simulink model "IEEE24bus"  (R2019b)
settings: Solver=VariableStepAuto  StartTime=0.0  StopTime=100  RelTol=1e-3
values from neighbouring files (symbols this model uses):
  C_b = 1/(w_b*Z_b)    (= 5.01433343075e-06)    [IEEE24_bus.m]
  Exc = [ 011	0	 200	0.02	1.12   0.5   0	0       0       0       0       0 ... (first row only)    [IEEE24_bus.m]
  G_data = [ 011	15.8 138	2.8	0.2     2.7	1.5     0.3     7.5     0.25	0.04	0.85	0.85	0.25	0.12	0 ... (first row only)    [IEEE24_bus.m]
  H011 = 4    [IEEE24_bus.m]
  H012 = 4    [IEEE24_bus.m]
  H013 = 4    [IEEE24_bus.m]
  H021 = 4    [IEEE24_bus.m]
  H022 = 4    [IEEE24_bus.m]
  H023 = 4    [IEEE24_bus.m]
  H024 = 4    [IEEE24_bus.m]
  H025 = 4    [IEEE24_bus.m]
  H026 = 4    [IEEE24_bus.m]
  H131 = 4    [IEEE24_bus.m]
  H132 = 4    [IEEE24_bus.m]
  H133 = 4    [IEEE24_bus.m]
  H134 = 4    [IEEE24_bus.m]
  H135 = 4    [IEEE24_bus.m]
  H151 = 4    [IEEE24_bus.m]
  H152 = 4    [IEEE24_bus.m]
  H153 = 4    [IEEE24_bus.m]
  H154 = 4    [IEEE24_bus.m]
  H161 = 4    [IEEE24_bus.m]
  H181 = 3.25    [IEEE24_bus.m]
  H211 = 4    [IEEE24_bus.m]
  H212 = 4    [IEEE24_bus.m]
  H213 = 4    [IEEE24_bus.m]
  H215 = 4    [IEEE24_bus.m]
  H216 = 4    [IEEE24_bus.m]
  H221 = 3.25    [IEEE24_bus.m]
  H231 = 4    [IEEE24_bus.m]
  H232 = 4    [IEEE24_bus.m]
  H233 = 4    [IEEE24_bus.m]
  H234 = 4    [IEEE24_bus.m]
  H235 = 4    [IEEE24_bus.m]
  L_b = Z_b/w_b    (= 1.40321608159)    [IEEE24_bus.m]
  PSSMODEL = 1    [IEEE24_bus.m]    (also in IEEE24bus_simplified_benchmark.m)
  Z_b = (V_b^2)/S_b    (= 529)    [IEEE24_bus.m]
undefined symbols (not defined in the file or in its folder): D1, Delta
libraries: powerlib x258, sps_avr x33, microgridLibrary x6
(part 1 of 6)
settings Model: SimulationMode=accelerator  Creator=mingj  LastModifiedBy=tmj89

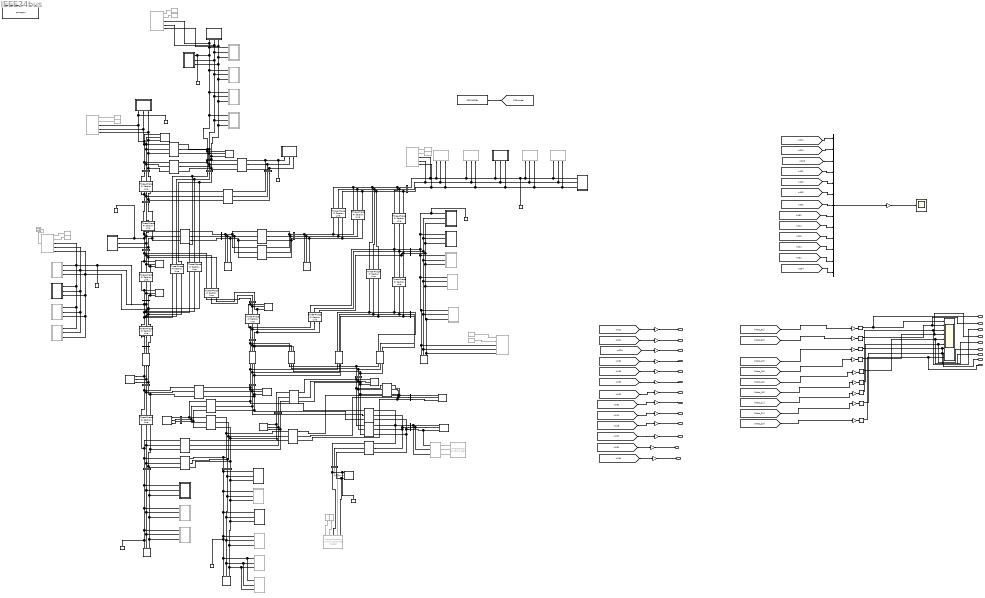
== system IEEE24bus ==
  011 : Subsystem
  012 : Subsystem  Commented=on
  013 : Subsystem  Commented=on
  "021 " : Subsystem
  022 : Subsystem  Commented=on
  023 : Subsystem
  024 : Subsystem  Commented=on
  025 : Subsystem  Commented=on
  026 : Subsystem  Commented=on
  1 : powerlib/Elements/Three-Phase PI Section Line  LConnTagsString=a|b|c  RConnTagsString=A|B|C  Frequency=60  Resistances="[0.00331*Z_b  0.00331*Z_b*3]"  Inductances="[0.02595*L_b  0.02595*L_b*3]"  Capacitances=[0.05330*C_b 0.05330*C_b/3]  Length=1
      settings: SourceProductName=Simscape Power Systems
  10 : powerlib/Elements/Three-Phase PI Section Line  LConnTagsString=a|b|c  RConnTagsString=A|B|C  Frequency=60  Resistances="[0.01224*Z_b  0.01224*Z_b*3]"  Inductances="[0.09644*L_b  0.09644*L_b*3]"  Capacitances=[0.1984*C_b 0.1984*C_b/3]  Length=1
      settings: SourceProductName=Simscape Power Systems
  11 : powerlib/Elements/Three-Phase PI Section Line  LConnTagsString=a|b|c  RConnTagsString=A|B|C  Frequency=60  Resistances="[0.01060*Z_b  0.01060*Z_b*3]"  Inductances="[0.08643*L_b  0.08643*L_b*3]"  Capacitances=[0.17520*C_b 0.17520*C_b/3]  Length=1
      settings: SourceProductName=Simscape Power Systems
  12 : powerlib/Elements/Three-Phase PI Section Line  LConnTagsString=a|b|c  RConnTagsString=A|B|C  Frequency=60  Resistances="[0.00583*Z_b  0.00583*Z_b*3]"  Inductances="[0.0476*L_b  0.0476*L_b*3]"  Capacitances=[0.0959*C_b 0.0959*C_b/3]  Length=1
      settings: SourceProductName=Simscape Power Systems
  131 : Subsystem
  132 : Subsystem
  133 : Subsystem  Commented=on
  134 : Subsystem  Commented=on
  135 : Subsystem  Commented=on
  14 : powerlib/Elements/Three-Phase PI Section Line  LConnTagsString=a|b|c  RConnTagsString=A|B|C  Frequency=60  Resistances="[0.00477*Z_b  0.00477*Z_b*3]"  Inductances="[0.03884*L_b  0.03884*L_b*3]"  Capacitances=[0.0785*C_b 0.0785*C_b/3]  Length=1
      settings: SourceProductName=Simscape Power Systems
  15 : powerlib/Elements/Three-Phase PI Section Line  LConnTagsString=a|b|c  RConnTagsString=A|B|C  Frequency=60  Resistances="[0.00513*Z_b  0.00513*Z_b*3]"  Inductances="[0.04172*L_b  0.04172*L_b*3]"  Capacitances=[0.0843*C_b 0.0843*C_b/3]  Length=1
      settings: SourceProductName=Simscape Power Systems
  151 : Subsystem  Commented=on
  152 : Subsystem
  153 : Subsystem  Commented=on
  154 : Subsystem  Commented=on
  16 : powerlib/Elements/Three-Phase PI Section Line  LConnTagsString=a|b|c  RConnTagsString=A|B|C  Frequency=60  Resistances="[0.00583*Z_b  0.00583*Z_b*3]"  Inductances="[0.04746*L_b  0.04746*L_b*3]"  Capacitances=[0.0959*C_b 0.0959*C_b/3]  Length=1
      settings: SourceProductName=Simscape Power Systems
  161 : Subsystem
  17 : powerlib/Elements/Three-Phase PI Section Line  LConnTagsString=a|b|c  RConnTagsString=A|B|C  Frequency=60  Resistances="[0.00642*Z_b  0.00642*Z_b*3]"  Inductances="[0.05187*L_b  0.05187*L_b*3]"  Capacitances=[0.1066*C_b 0.1066*C_b/3]  Length=1
      settings: SourceProductName=Simscape Power Systems
  18 : powerlib/Elements/Three-Phase PI Section Line  LConnTagsString=a|b|c  RConnTagsString=A|B|C  Frequency=60  Resistances="[0.05419*Z_b  0.05419*Z_b*3]"  Inductances="[0.21114*L_b  0.21114*L_b*3]"  Capacitances=[0.0613*C_b 0.0613*C_b/3]  Length=1
      settings: SourceProductName=Simscape Power Systems
  181 : Subsystem
  19 : powerlib/Elements/Three-Phase PI Section Line  LConnTagsString=a|b|c  RConnTagsString=A|B|C  Frequency=60  Resistances="[0.002*Z_b  0.002*Z_b*3]"  Inductances="[0.119*L_b  0.119*L_b*3]"  Capacitances=[0.0343*C_b 0.0343*C_b/3]  Length=1
      settings: SourceProductName=Simscape Power Systems
  2 : powerlib/Elements/Three-Phase PI Section Line  LConnTagsString=a|b|c  RConnTagsString=A|B|C  Frequency=60  Resistances="[0.00331*Z_b  0.00331*Z_b*3]"  Inductances="[0.02595*L_b  0.02595*L_b*3]"  Capacitances=[0.05330*C_b 0.05330*C_b/3]  Length=1
      settings: SourceProductName=Simscape Power Systems
  20 : powerlib/Elements/Three-Phase PI Section Line  LConnTagsString=a|b|c  RConnTagsString=A|B|C  Frequency=60  Resistances="[0.002*Z_b  0.002*Z_b*3]"  Inductances=[0.088*L_b 0.088*L_b*3]  Capacitances=[0.0478*C_b 0.0478*C_b/3]  Length=1
      settings: SourceProductName=Simscape Power Systems
  21 : powerlib/Elements/Three-Phase PI Section Line  LConnTagsString=a|b|c  RConnTagsString=A|B|C  Frequency=60  Resistances="[0.02692*Z_b  0.02692*Z_b*3]"  Inductances="[0.10779*L_b  0.10779*L_b*3]"  Capacitances=[0.0279*C_b 0.0279*C_b/3]  Length=1
      settings: SourceProductName=Simscape Power Systems
  211 : Subsystem
  212 : Subsystem  Commented=on
  213 : Subsystem  Commented=on
  214 : Subsystem  Commented=on
  215 : Subsystem  Commented=on
  216 : Subsystem
  22 : powerlib/Elements/Three-Phase PI Section Line  LConnTagsString=a|b|c  RConnTagsString=A|B|C  Frequency=60  Resistances=[0.03361*Z_b 0.03361*Z_b*3]  Inductances="[0.1273*L_b  0.1273*L_b*3]"  Capacitances=[0.0366*C_b 0.0366*C_b/3]  Length=1
      settings: SourceProductName=Simscape Power Systems
  221 : Subsystem
  23 : powerlib/Elements/Three-Phase PI Section Line  LConnTagsString=a|b|c  RConnTagsString=A|B|C  Frequency=60  Resistances="[0.02243*Z_b  0.02243*Z_b*3]"  Inductances=[0.0849*L_b 0.0849*L_b*3]  Capacitances=[0.0849*C_b 0.0849*C_b/3]  Length=1
      settings: SourceProductName=Simscape Power Systems
  231 : Subsystem
  232 : Subsystem  Commented=on
  233 : Subsystem  Commented=on
  234 : Subsystem
  235 : Subsystem  Commented=on
  236 : Subsystem  Commented=on
  24 : powerlib/Elements/Three-Phase PI Section Line  LConnTagsString=a|b|c  RConnTagsString=A|B|C  Frequency=60  Resistances="[0.0025*Z_b  0.0025*Z_b*3]"  Inductances="[0.014*L_b  0.014*L_b*3]"  Capacitances=[0.00065*C_b 0.00065*C_b/3]  Length=1
      settings: SourceProductName=Simscape Power Systems
  25 : powerlib/Elements/Three-Phase PI Section Line  LConnTagsString=a|b|c  RConnTagsString=A|B|C  Frequency=60  Resistances="[0.00607*Z_b  0.00607*Z_b*3]"  Inductances="[0.04899*L_b  0.04899*L_b*3]"  Capacitances=[0.10060*C_b 0.10060*C_b/3]  Length=1
      settings: SourceProductName=Simscape Power Systems
  26 : powerlib/Elements/Three-Phase PI Section Line  LConnTagsString=a|b|c  RConnTagsString=A|B|C  Frequency=60  Resistances="[0.05064*Z_b  0.05064*Z_b*3]"  Inductances="[0.19201*L_b  0.19201*L_b*3]"  Capacitances=[0.0557*C_b 0.0557*C_b/3]  Length=1
      settings: SourceProductName=Simscape Power Systems
  27 : powerlib/Elements/Three-Phase PI Section Line  LConnTagsString=a|b|c  RConnTagsString=A|B|C  Frequency=60  Resistances="[0.02262*Z_b  0.02262*Z_b*3]"  Inductances="[0.03333*L_b  0.03333*L_b*3]"  Capacitances=[0.13029*C_b 0.13029*C_b/3]  Length=1
      settings: SourceProductName=Simscape Power Systems
  28 : powerlib/Elements/Three-Phase PI Section Line  LConnTagsString=a|b|c  RConnTagsString=A|B|C  Frequency=60  Resistances="[0.00318*Z_b  0.00318*Z_b*3]"  Inductances="[0.025920*L_b  0.025920*L_b*3]"  Capacitances=[0.05230*C_b 0.05230*C_b/3]  Length=1
      settings: SourceProductName=Simscape Power Systems
  29 : powerlib/Elements/Three-Phase PI Section Line  LConnTagsString=a|b|c  RConnTagsString=A|B|C  Frequency=60  Resistances="[0.04234*Z_b  0.04234*Z_b*3]"  Inductances="[0.16482*L_b  0.16482*L_b*3]"  Capacitances=[0.0478*C_b 0.0478*C_b/3]  Length=1
      settings: SourceProductName=Simscape Power Systems
  3 : powerlib/Elements/Three-Phase PI Section Line  LConnTagsString=a|b|c  RConnTagsString=A|B|C  Frequency=60  Resistances="[0.00829*Z_b  0.00829*Z_b*3]"  Inductances="[0.06769*L_b  0.06769*L_b*3]"  Capacitances=[0.13670*C_b 0.13670*C_b/3]  Length=1
      settings: SourceProductName=Simscape Power Systems
  3-Phase Dynamic Load3 : powerlib/Elements/Three-Phase Dynamic Load  Commented=on  NominalVoltage=[ 20e3 60 ]  ActiveReactivePowers=[-1e6 -1e6]  PositiveSequence=[0.999196 -2.87767]  ExternalControl=off  NpNq="[0  0]"  TimeConstants=[0 0 0 0]  MinimumVoltage=0.01  Tfilter=1e-1  LoadFlowParameters=[4 50000000 0 0 25000000]
      settings: SourceProductName=Simscape Power Systems  SourceProductBaseCode=PS
  30 : powerlib/Elements/Three-Phase PI Section Line  LConnTagsString=a|b|c  RConnTagsString=A|B|C  Frequency=60  Resistances="[0.00177*Z_b  0.00177*Z_b*3]"  Inductances="[0.01439*L_b  0.01439*L_b*3]"  Capacitances=[0.02910*C_b 0.02910*C_b/3]  Length=1
      settings: SourceProductName=Simscape Power Systems
  31 : powerlib/Elements/Three-Phase PI Section Line  LConnTagsString=a|b|c  RConnTagsString=A|B|C  Frequency=60  Resistances="[0.04234*Z_b  0.04234*Z_b*3]"  Inductances="[0.16482*L_b  0.16482*L_b*3]"  Capacitances=[0.0478*C_b 0.0478*C_b/3]  Length=1
      settings: SourceProductName=Simscape Power Systems
  32 : powerlib/Elements/Three-Phase PI Section Line  LConnTagsString=a|b|c  RConnTagsString=A|B|C  Frequency=60  Resistances=[0.01614*Z_b 0.01614*Z_b*3]  Inductances="[0.06103*L_b  0.06103*L_b*3]"  Capacitances=[0.0179*C_b 0.0179*C_b/3]  Length=1
      settings: SourceProductName=Simscape Power Systems
  4 : powerlib/Elements/Three-Phase PI Section Line  LConnTagsString=a|b|c  RConnTagsString=A|B|C  Frequency=60  Resistances="[0.01225*Z_b  0.01225*Z_b*3]"  Inductances="[0.10527*L_b  0.10527*L_b*3]"  Capacitances=[0.21160*C_b 0.21160*C_b/3]  Length=1
      settings: SourceProductName=Simscape Power Systems
  43 : powerlib/Elements/Three-Phase PI Section Line  LConnTagsString=a|b|c  RConnTagsString=A|B|C  Frequency=60  Resistances=[0.00607*Z_b 0.00607*Z_b*3]  Inductances="[0.04899*L_b  0.04899*L_b*3]"  Capacitances=[0.10060*C_b 0.10060*C_b/3]  Length=1
      settings: SourceProductName=Simscape Power Systems
  5 : powerlib/Elements/Three-Phase PI Section Line  LConnTagsString=a|b|c  RConnTagsString=A|B|C  Frequency=60  Resistances="[0.00283*Z_b  0.00283*Z_b*3]"  Inductances="[0.02302*L_b  0.02302*L_b*3]"  Capacitances=[0.04650*C_b 0.04650*C_b/3]  Length=1
      settings: SourceProductName=Simscape Power Systems
  6 : powerlib/Elements/Three-Phase PI Section Line  LConnTagsString=a|b|c  RConnTagsString=A|B|C  Frequency=60  Resistances="[0.00505*Z_b  0.00505*Z_b*3]"  Inductances="[0.03964*L_b  0.03964*L_b*3]"  Capacitances=[0.08140*C_b 0.08140*C_b/3]  Length=1
      settings: SourceProductName=Simscape Power Systems
  7 : powerlib/Elements/Three-Phase PI Section Line  LConnTagsString=a|b|c  RConnTagsString=A|B|C  Frequency=60  Resistances="[0.00505*Z_b  0.00505*Z_b*3]"  Inductances="[0.03964*L_b  0.03964*L_b*3]"  Capacitances=[0.08140*C_b 0.08140*C_b/3]  Length=1
      settings: SourceProductName=Simscape Power Systems
  8 : powerlib/Elements/Three-Phase PI Section Line  LConnTagsString=a|b|c  RConnTagsString=A|B|C  Frequency=60  Resistances="[0.00276*Z_b  0.00276*Z_b*3]"  Inductances="[0.02163*L_b  0.02163*L_b*3]"  Capacitances=[0.04440*C_b 0.04440*C_b/3]  Length=1
      settings: SourceProductName=Simscape Power Systems
  9 : powerlib/Elements/Three-Phase PI Section Line  LConnTagsString=a|b|c  RConnTagsString=A|B|C  Frequency=60  Resistances="[0.00276*Z_b  0.00276*Z_b*3]"  Inductances="[0.02163*L_b  0.02163*L_b*3]"  Capacitances=[0.04440*C_b 0.04440*C_b/3]  Length=1
      settings: SourceProductName=Simscape Power Systems
  Base Load 1 : powerlib/Elements/Three-Phase Parallel RLC Load  LConnTagsString=A|B|C  Configuration=Y (grounded)  NominalVoltage=230e3  Vabc=[1e3 1e3 1e3]  Vabcp=[1e3 1e3 1e3]  NominalFrequency=60  UnbalancedPower=off  ActivePower=L19  InductivePower=18e6  CapacitivePower=0  Pabc=[10e3 9e3 11e3]  QLabc=[100 90 110]  QCabc=[100 90 110]  Pabcp=[10e3 9e3 11e3]  QLabcp=[100 90 110]  QCabcp=[100 90 110]  Measurements=None  LoadType=constant Z
      settings: SourceProductName=Simscape Electrical
  Base Load 10 : powerlib/Elements/Three-Phase Parallel RLC Load  LConnTagsString=A|B|C  Configuration=Y (grounded)  NominalVoltage=138e3  Vabc=[1e3 1e3 1e3]  Vabcp=[1e3 1e3 1e3]  NominalFrequency=60  UnbalancedPower=off  ActivePower=L1  InductivePower=22e6  CapacitivePower=0  Pabc=[10e3 9e3 11e3]  QLabc=[100 90 110]  QCabc=[100 90 110]  Pabcp=[10e3 9e3 11e3]  QLabcp=[100 90 110]  QCabcp=[100 90 110]  Measurements=None  LoadType=constant Z
      settings: SourceProductName=Simscape Electrical
  Base Load 11 : powerlib/Elements/Three-Phase Parallel RLC Load  LConnTagsString=A|B|C  Configuration=Y (grounded)  NominalVoltage=138e3  Vabc=[1e3 1e3 1e3]  Vabcp=[1e3 1e3 1e3]  NominalFrequency=60  UnbalancedPower=off  ActivePower=L2  InductivePower=20e6  CapacitivePower=0  Pabc=[10e3 9e3 11e3]  QLabc=[100 90 110]  QCabc=[100 90 110]  Pabcp=[10e3 9e3 11e3]  QLabcp=[100 90 110]  QCabcp=[100 90 110]  Measurements=None  LoadType=constant Z
      settings: SourceProductName=Simscape Electrical
  Base Load 12 : powerlib/Elements/Three-Phase Parallel RLC Load  LConnTagsString=A|B|C  Configuration=Y (grounded)  NominalVoltage=138e3  Vabc=[1e3 1e3 1e3]  Vabcp=[1e3 1e3 1e3]  NominalFrequency=60  UnbalancedPower=off  ActivePower=L3  InductivePower=19e6  CapacitivePower=0  Pabc=[10e3 9e3 11e3]  QLabc=[100 90 110]  QCabc=[100 90 110]  Pabcp=[10e3 9e3 11e3]  QLabcp=[100 90 110]  QCabcp=[100 90 110]  Measurements=None  LoadType=constant Z
      settings: SourceProductName=Simscape Electrical
  Base Load 13 : powerlib/Elements/Three-Phase Parallel RLC Load  LConnTagsString=A|B|C  Configuration=Y (grounded)  NominalVoltage=138e3  Vabc=[1e3 1e3 1e3]  Vabcp=[1e3 1e3 1e3]  NominalFrequency=60  UnbalancedPower=off  ActivePower=L5  InductivePower=14e6  CapacitivePower=0  Pabc=[10e3 9e3 11e3]  QLabc=[100 90 110]  QCabc=[100 90 110]  Pabcp=[10e3 9e3 11e3]  QLabcp=[100 90 110]  QCabcp=[100 90 110]  Measurements=None  LoadType=constant Z
      settings: SourceProductName=Simscape Electrical
  Base Load 14 : powerlib/Elements/Three-Phase Parallel RLC Load  LConnTagsString=A|B|C  Configuration=Y (grounded)  NominalVoltage=230e3  Vabc=[1e3 1e3 1e3]  Vabcp=[1e3 1e3 1e3]  NominalFrequency=60  UnbalancedPower=off  ActivePower=L13  InductivePower=27e6  CapacitivePower=0  Pabc=[10e3 9e3 11e3]  QLabc=[100 90 110]  QCabc=[100 90 110]  Pabcp=[10e3 9e3 11e3]  QLabcp=[100 90 110]  QCabcp=[100 90 110]  Measurements=None  LoadType=constant Z
      settings: SourceProductName=Simscape Electrical
  Base Load 15 : powerlib/Elements/Three-Phase Parallel RLC Load  LConnTagsString=A|B|C  Configuration=Y (grounded)  NominalVoltage=230e3  Vabc=[1e3 1e3 1e3]  Vabcp=[1e3 1e3 1e3]  NominalFrequency=60  UnbalancedPower=off  ActivePower=L14  InductivePower=20e6  CapacitivePower=0  Pabc=[10e3 9e3 11e3]  QLabc=[100 90 110]  QCabc=[100 90 110]  Pabcp=[10e3 9e3 11e3]  QLabcp=[100 90 110]  QCabcp=[100 90 110]  Measurements=None  LoadType=constant Z
      settings: SourceProductName=Simscape Electrical
  Base Load 16 : powerlib/Elements/Three-Phase Parallel RLC Load  LConnTagsString=A|B|C  Configuration=Y (grounded)  NominalVoltage=230e3  Vabc=[1e3 1e3 1e3]  Vabcp=[1e3 1e3 1e3]  NominalFrequency=60  UnbalancedPower=off  ActivePower=L15  InductivePower=32e6  CapacitivePower=0  Pabc=[10e3 9e3 11e3]  QLabc=[100 90 110]  QCabc=[100 90 110]  Pabcp=[10e3 9e3 11e3]  QLabcp=[100 90 110]  QCabcp=[100 90 110]  Measurements=None  LoadType=constant Z
      settings: SourceProductName=Simscape Electrical
  Base Load 17 : powerlib/Elements/Three-Phase Parallel RLC Load  LConnTagsString=A|B|C  Configuration=Y (grounded)  NominalVoltage=230e3  Vabc=[1e3 1e3 1e3]  Vabcp=[1e3 1e3 1e3]  NominalFrequency=60  UnbalancedPower=off  ActivePower=L16  InductivePower=0  CapacitivePower=0  Pabc=[10e3 9e3 11e3]  QLabc=[100 90 110]  QCabc=[100 90 110]  Pabcp=[10e3 9e3 11e3]  QLabcp=[100 90 110]  QCabcp=[100 90 110]  Measurements=None  LoadType=constant Z
      settings: SourceProductName=Simscape Electrical
  Base Load 18 : powerlib/Elements/Three-Phase Parallel RLC Load  LConnTagsString=A|B|C  Configuration=Y (grounded)  NominalVoltage=230e3  Vabc=[1e3 1e3 1e3]  Vabcp=[1e3 1e3 1e3]  NominalFrequency=60  UnbalancedPower=off  ActivePower=L21  InductivePower=34e6  CapacitivePower=0  Pabc=[10e3 9e3 11e3]  QLabc=[100 90 110]  QCabc=[100 90 110]  Pabcp=[10e3 9e3 11e3]  QLabcp=[100 90 110]  QCabcp=[100 90 110]  Measurements=None  LoadType=constant Z
      settings: SourceProductName=Simscape Electrical
  Base Load 2 : powerlib/Elements/Three-Phase Parallel RLC Load  LConnTagsString=A|B|C  Configuration=Y (grounded)  NominalVoltage=230e3  Vabc=[1e3 1e3 1e3]  Vabcp=[1e3 1e3 1e3]  NominalFrequency=60  UnbalancedPower=off  ActivePower=L20  InductivePower=13e6  CapacitivePower=0  Pabc=[10e3 9e3 11e3]  QLabc=[100 90 110]  QCabc=[100 90 110]  Pabcp=[10e3 9e3 11e3]  QLabcp=[100 90 110]  QCabcp=[100 90 110]  Measurements=None  LoadType=constant Z
      settings: SourceProductName=Simscape Electrical
  Base Load 3 : powerlib/Elements/Three-Phase Parallel RLC Load  LConnTagsString=A|B|C  Configuration=Y (grounded)  NominalVoltage=138e3  Vabc=[1e3 1e3 1e3]  Vabcp=[1e3 1e3 1e3]  NominalFrequency=60  UnbalancedPower=off  ActivePower=L6  InductivePower=14e6  CapacitivePower=0  Pabc=[10e3 9e3 11e3]  QLabc=[100 90 110]  QCabc=[100 90 110]  Pabcp=[10e3 9e3 11e3]  QLabcp=[100 90 110]  QCabcp=[100 90 110]  Measurements=None  LoadType=constant Z
      settings: SourceProductName=Simscape Electrical
  Base Load 4 : powerlib/Elements/Three-Phase Parallel RLC Load  LConnTagsString=A|B|C  Configuration=Y (grounded)  NominalVoltage=138e3  Vabc=[1e3 1e3 1e3]  Vabcp=[1e3 1e3 1e3]  NominalFrequency=60  UnbalancedPower=off  ActivePower=L8  InductivePower=18e6  CapacitivePower=0  Pabc=[10e3 9e3 11e3]  QLabc=[100 90 110]  QCabc=[100 90 110]  Pabcp=[10e3 9e3 11e3]  QLabcp=[100 90 110]  QCabcp=[100 90 110]  Measurements=None  LoadType=constant Z
      settings: SourceProductName=Simscape Electrical
  Base Load 5 : powerlib/Elements/Three-Phase Parallel RLC Load  LConnTagsString=A|B|C  Configuration=Y (grounded)  NominalVoltage=230e3  Vabc=[1e3 1e3 1e3]  Vabcp=[1e3 1e3 1e3]  NominalFrequency=60  UnbalancedPower=off  ActivePower=L18  InductivePower=34e6  CapacitivePower=0  Pabc=[10e3 9e3 11e3]  QLabc=[100 90 110]  QCabc=[100 90 110]  Pabcp=[10e3 9e3 11e3]  QLabcp=[100 90 110]  QCabcp=[100 90 110]  Measurements=None  LoadType=constant Z
      settings: SourceProductName=Simscape Electrical
  Base Load 6 : powerlib/Elements/Three-Phase Parallel RLC Load  LConnTagsString=A|B|C  Configuration=Y (grounded)  NominalVoltage=138e3  Vabc=[1e3 1e3 1e3]  Vabcp=[1e3 1e3 1e3]  NominalFrequency=60  UnbalancedPower=off  ActivePower=L4  InductivePower=15e6  CapacitivePower=0  Pabc=[10e3 9e3 11e3]  QLabc=[100 90 110]  QCabc=[100 90 110]  Pabcp=[10e3 9e3 11e3]  QLabcp=[100 90 110]  QCabcp=[100 90 110]  Measurements=None  LoadType=constant Z
      settings: SourceProductName=Simscape Electrical
  Base Load 7 : powerlib/Elements/Three-Phase Parallel RLC Load  LConnTagsString=A|B|C  Configuration=Y (grounded)  NominalVoltage=138e3  Vabc=[1e3 1e3 1e3]  Vabcp=[1e3 1e3 1e3]  NominalFrequency=60  UnbalancedPower=off  ActivePower=L9  InductivePower=36e6  CapacitivePower=0  Pabc=[10e3 9e3 11e3]  QLabc=[100 90 110]  QCabc=[100 90 110]  Pabcp=[10e3 9e3 11e3]  QLabcp=[100 90 110]  QCabcp=[100 90 110]  Measurements=None  LoadType=constant Z
      settings: SourceProductName=Simscape Electrical
  Base Load 8 : powerlib/Elements/Three-Phase Parallel RLC Load  LConnTagsString=A|B|C  Configuration=Y (grounded)  NominalVoltage=138e3  Vabc=[1e3 1e3 1e3]  Vabcp=[1e3 1e3 1e3]  NominalFrequency=60  UnbalancedPower=off  ActivePower=L10  InductivePower=23e6  CapacitivePower=0  Pabc=[10e3 9e3 11e3]  QLabc=[100 90 110]  QCabc=[100 90 110]  Pabcp=[10e3 9e3 11e3]  QLabcp=[100 90 110]  QCabcp=[100 90 110]  Measurements=None  LoadType=constant Z
      settings: SourceProductName=Simscape Electrical
  Base Load 9 : powerlib/Elements/Three-Phase Parallel RLC Load  LConnTagsString=A|B|C  Configuration=Y (grounded)  NominalVoltage=138e3  Vabc=[1e3 1e3 1e3]  Vabcp=[1e3 1e3 1e3]  NominalFrequency=60  UnbalancedPower=off  ActivePower=L7  InductivePower=13e6  CapacitivePower=0  Pabc=[10e3 9e3 11e3]  QLabc=[100 90 110]  QCabc=[100 90 110]  Pabcp=[10e3 9e3 11e3]  QLabcp=[100 90 110]  QCabcp=[100 90 110]  Measurements=None  LoadType=constant Z
      settings: SourceProductName=Simscape Electrical
  Bus1 : powerlib/Measurements/Three-Phase V-I Measurement  VoltageMeasurement=phase-to-phase  SetLabelV=on  LabelV=Vabc_01  Vpu=on  VpuLL=off  CurrentMeasurement=no  SetLabelI=on  LabelI=Iabc_1  Ipu=on  Pbase=S_b  Vbase=V_bl  OutputType=Complex  PhasorSimulation=on  PSBequivalent=0
      settings: SourceProductName=Simscape Electrical
  Bus{3..6,8..12,14,17,19,24} (13 alike) : powerlib/Measurements/Three-Phase V-I Measurement  VoltageMeasurement=no  SetLabelV=on  LabelV=Vabc_1  Vpu=on  VpuLL=off  CurrentMeasurement=no  SetLabelI=on  LabelI=Iabc_1  Ipu=on  Pbase=S_b  Vbase=V_b  OutputType=Complex  PhasorSimulation=on  PSBequivalent=0
      settings: SourceProductName=Simscape Electrical
  Bus13 : powerlib/Measurements/Three-Phase V-I Measurement  VoltageMeasurement=phase-to-phase  SetLabelV=on  LabelV=Vabc_13  Vpu=on  VpuLL=off  CurrentMeasurement=no  SetLabelI=on  LabelI=Iabc_1  Ipu=on  Pbase=S_b  Vbase=V_b  OutputType=Complex  PhasorSimulation=on  PSBequivalent=0
      settings: SourceProductName=Simscape Electrical
  Bus15 : powerlib/Measurements/Three-Phase V-I Measurement  VoltageMeasurement=phase-to-phase  SetLabelV=on  LabelV=Vabc_15  Vpu=on  VpuLL=off  CurrentMeasurement=no  SetLabelI=on  LabelI=Iabc_1  Ipu=on  Pbase=S_b  Vbase=V_b  OutputType=Complex  PhasorSimulation=on  PSBequivalent=0
      settings: SourceProductName=Simscape Electrical
  Bus16 : powerlib/Measurements/Three-Phase V-I Measurement  VoltageMeasurement=phase-to-phase  SetLabelV=on  LabelV=Vabc_16  Vpu=on  VpuLL=off  CurrentMeasurement=no  SetLabelI=on  LabelI=Iabc_1  Ipu=on  Pbase=S_b  Vbase=V_b  OutputType=Complex  PhasorSimulation=on  PSBequivalent=0
      settings: SourceProductName=Simscape Electrical
  Bus18 : powerlib/Measurements/Three-Phase V-I Measurement  VoltageMeasurement=phase-to-phase  SetLabelV=on  LabelV=Vabc_18  Vpu=on  VpuLL=off  CurrentMeasurement=no  SetLabelI=on  LabelI=Iabc_1  Ipu=on  Pbase=S_b  Vbase=V_b  OutputType=Complex  PhasorSimulation=on  PSBequivalent=0
      settings: SourceProductName=Simscape Electrical
  Bus2 : powerlib/Measurements/Three-Phase V-I Measurement  VoltageMeasurement=phase-to-phase  SetLabelV=on  LabelV=Vabc_02  Vpu=on  VpuLL=off  CurrentMeasurement=no  SetLabelI=on  LabelI=Iabc_1  Ipu=on  Pbase=S_b  Vbase=V_bl  OutputType=Complex  PhasorSimulation=on  PSBequivalent=0
      settings: SourceProductName=Simscape Electrical
  Bus20 : powerlib/Measurements/Three-Phase V-I Measurement  VoltageMeasurement=no  SetLabelV=on  LabelV=Vabc_20  Vpu=on  VpuLL=off  CurrentMeasurement=yes  SetLabelI=on  LabelI=Iabc_20  Ipu=on  Pbase=S_b  Vbase=V_b  OutputType=Complex  PhasorSimulation=on  PSBequivalent=0
      settings: SourceProductName=Simscape Electrical
  Bus21 : powerlib/Measurements/Three-Phase V-I Measurement  VoltageMeasurement=phase-to-phase  SetLabelV=on  LabelV=Vabc_21  Vpu=on  VpuLL=off  CurrentMeasurement=no  SetLabelI=on  LabelI=Iabc_1  Ipu=on  Pbase=S_b  Vbase=V_b  OutputType=Complex  PhasorSimulation=on  PSBequivalent=0
      settings: SourceProductName=Simscape Electrical
  Bus22 : powerlib/Measurements/Three-Phase V-I Measurement  VoltageMeasurement=phase-to-phase  SetLabelV=on  LabelV=Vabc_22  Vpu=on  VpuLL=off  CurrentMeasurement=no  SetLabelI=on  LabelI=Iabc_1  Ipu=on  Pbase=S_b  Vbase=V_b  OutputType=Complex  PhasorSimulation=on  PSBequivalent=0
      settings: SourceProductName=Simscape Electrical
  Bus23 : powerlib/Measurements/Three-Phase V-I Measurement  VoltageMeasurement=phase-to-phase  SetLabelV=on  LabelV=Vabc_23  Vpu=on  VpuLL=off  CurrentMeasurement=no  SetLabelI=on  LabelI=Iabc_1  Ipu=on  Pbase=S_b  Vbase=V_b  OutputType=Complex  PhasorSimulation=on  PSBequivalent=0
      settings: SourceProductName=Simscape Electrical
  Bus7 : powerlib/Measurements/Three-Phase V-I Measurement  VoltageMeasurement=phase-to-phase  SetLabelV=on  LabelV=Vabc_07  Vpu=on  VpuLL=off  CurrentMeasurement=no  SetLabelI=on  LabelI=Iabc_1  Ipu=on  Pbase=S_b  Vbase=V_bl  OutputType=Complex  PhasorSimulation=on  PSBequivalent=0
      settings: SourceProductName=Simscape Electrical
  CPS mag : Scope  NumInputPorts=9
  Constant{8,10,13,19,25,27} (6 alike) : Constant  Commented=on  Value=0
  Constant{9,11,14,20,26,28} (6 alike) : Constant  Commented=on  Value=15
  Gain{,1..8} (9 alike) : Gain  Gain=[1 0 0]  Multiplication=Matrix(K*u) (u vector)
  L-49-2 : powerlib/Elements/Three-Phase PI Section Line  LConnTagsString=a|b|c  RConnTagsString=A|B|C  Frequency=60  Resistances="[0.00212*Z_b  0.00212*Z_b*3]"  Inductances="[ 0.17269*L_b  0.17269*L_b*3]"  Capacitances=[ 0.03490*C_b 0.03490*C_b/3]  Length=1
      settings: SourceProductName=Simscape Power Systems
  Load Flow Bus : powerlib/Measurements/Load Flow Bus  LConnTagsString=a  Phases=single  Connectors=on one side  ID=BUS_18  Vbase=230e3  Vref=1.05  Vangle=0  VLF=0.975  VLFb=1  VLFc=1  angleLF=48.06  angleLFb=0  angleLFc=0
      settings: AttributesFormatString=%<ID>\n%<Vbase>V\n%<VLF>pu\n%<angleLF>deg.  SourceProductName=Simscape Electrical
  Load Flow Bus1 : powerlib/Measurements/Load Flow Bus  LConnTagsString=a  Phases=single  Connectors=on one side  ID=BUS_02  Vbase=138e3  Vref=1.035  Vangle=0  VLF=1.001  VLFb=1  VLFc=1  angleLF=21.1  angleLFb=0  angleLFc=0
      settings: AttributesFormatString=%<ID>\n%<Vbase>V\n%<VLF>pu\n%<angleLF>deg.  SourceProductName=Simscape Electrical
  Load Flow Bus10 : powerlib/Measurements/Load Flow Bus  LConnTagsString=a  Phases=single  Connectors=on one side  ID=BUS_13  Vbase=230e3  Vref=1.02  Vangle=0  VLF=0.9742  VLFb=1  VLFc=1  angleLF=29.58  angleLFb=0  angleLFc=0
      settings: AttributesFormatString=%<ID>\n%<Vbase>V\n%<VLF>pu\n%<angleLF>deg.  SourceProductName=Simscape Electrical
  Load Flow Bus11 : powerlib/Measurements/Load Flow Bus  LConnTagsString=a  Phases=single  Connectors=on one side  ID=BUS_16  Vbase=230e3  Vref=1.017  Vangle=0  VLF=0.9617  VLFb=1  VLFc=1  angleLF=41.74  angleLFb=0  angleLFc=0
      settings: AttributesFormatString=%<ID>\n%<Vbase>V\n%<VLF>pu\n%<angleLF>deg.  SourceProductName=Simscape Electrical
  Load Flow Bus2 : powerlib/Measurements/Load Flow Bus  LConnTagsString=a  Phases=single  Connectors=on one side  ID=BUS_07  Vbase=138e3  Vref=1.025  Vangle=0  VLF=0.9748  VLFb=1  VLFc=1  angleLF=21.22  angleLFb=0  angleLFc=0
      settings: AttributesFormatString=%<ID>\n%<Vbase>V\n%<VLF>pu\n%<angleLF>deg.  SourceProductName=Simscape Electrical
  Load Flow Bus3 : powerlib/Measurements/Load Flow Bus  LConnTagsString=a  Phases=single  Connectors=on one side  ID=BUS_21  Vbase=230e3  Vref=1.05  Vangle=0  VLF=0.9792  VLFb=1  VLFc=1  angleLF=48.86  angleLFb=0  angleLFc=0
      settings: AttributesFormatString=%<ID>\n%<Vbase>V\n%<VLF>pu\n%<angleLF>deg.  SourceProductName=Simscape Electrical
  Load Flow Bus4 : powerlib/Measurements/Load Flow Bus  LConnTagsString=a  Phases=single  Connectors=on one side  ID=BUS_01  Vbase=138e3  Vref=1.035  Vangle=0  VLF=0.9978  VLFb=1  VLFc=1  angleLF=21.25  angleLFb=0  angleLFc=0
      settings: AttributesFormatString=%<ID>\n%<Vbase>V\n%<VLF>pu\n%<angleLF>deg.  SourceProductName=Simscape Electrical
  Load Flow Bus5 : powerlib/Measurements/Load Flow Bus  LConnTagsString=a  Phases=single  Connectors=on one side  ID=BUS_15  Vbase=230e3  Vref=1.014  Vangle=0  VLF=0.9593  VLFb=1  VLFc=1  angleLF=42.73  angleLFb=0  angleLFc=0
      settings: AttributesFormatString=%<ID>\n%<Vbase>V\n%<VLF>pu\n%<angleLF>deg.  SourceProductName=Simscape Electrical
  Load Flow Bus6 : powerlib/Measurements/Load Flow Bus  LConnTagsString=a  Phases=single  Connectors=on one side  ID=BUS_22  Vbase=230e3  Vref=1.05  Vangle=0  VLF=0.9939  VLFb=1  VLFc=1  angleLF=55.21  angleLFb=0  angleLFc=0
      settings: AttributesFormatString=%<ID>\n%<Vbase>V\n%<VLF>pu\n%<angleLF>deg.  SourceProductName=Simscape Electrical
  Load Flow Bus7 : powerlib/Measurements/Load Flow Bus  LConnTagsString=a  Phases=single  Connectors=on one side  ID=BUS_23  Vbase=230e3  Vref=1.05  Vangle=0  VLF=0.9824  VLFb=1  VLFc=1  angleLF=41.99  angleLFb=0  angleLFc=0
      settings: AttributesFormatString=%<ID>\n%<Vbase>V\n%<VLF>pu\n%<angleLF>deg.  SourceProductName=Simscape Electrical
  Mux : Mux  Inputs=13
  PSS model : Constant  Value=PSSMODEL
  Power Equation Wind Turbine (PQ Model)10 : microgridLibrary/Power Equation Wind Turbine (PQ Model)  Commented=on  Unom=15  Umax=25  Umin=5  Pselect=Simple Cubic Power  Vrms=230*1e3  Fnom=60  rp=5  Cp=16/27  rho=1.225  Pnom=60*1e6  Uvec=[1:1:30]  Pvec=[0,0,0,0,21359.3750000000,58193.5000000000,104316.125000000,157104.500000000,213935.875000000,272187.500000000,329236.625000000,382460.500000000,429236.375000000,466941.500000000,492953.125000000,500000,500000,500000,500000,500000,500000,500000,500000,500000,500000,0,0,0,0,0]  Tp=0.1  Tq=1  ReactP=0
  Power Equation Wind Turbine (PQ Model)11 : microgridLibrary/Power Equation Wind Turbine (PQ Model)  Commented=on  Unom=15  Umax=25  Umin=5  Pselect=Simple Cubic Power  Vrms=138*1e3  Fnom=60  rp=5  Cp=16/27  rho=1.225  Pnom=50e6  Uvec=[1:1:30]  Pvec=[0,0,0,0,21359.3750000000,58193.5000000000,104316.125000000,157104.500000000,213935.875000000,272187.500000000,329236.625000000,382460.500000000,429236.375000000,466941.500000000,492953.125000000,500000,500000,500000,500000,500000,500000,500000,500000,500000,500000,0,0,0,0,0]  Tp=0.1  Tq=1  ReactP=0
  Power Equation Wind Turbine (PQ Model)12 : microgridLibrary/Power Equation Wind Turbine (PQ Model)  Commented=on  Unom=15  Umax=25  Umin=5  Pselect=Simple Cubic Power  Vrms=230*1e3  Fnom=60  rp=5  Cp=16/27  rho=1.225  Pnom=160e6  Uvec=[1:1:30]  Pvec=[0,0,0,0,21359.3750000000,58193.5000000000,104316.125000000,157104.500000000,213935.875000000,272187.500000000,329236.625000000,382460.500000000,429236.375000000,466941.500000000,492953.125000000,500000,500000,500000,500000,500000,500000,500000,500000,500000,500000,0,0,0,0,0]  Tp=0.1  Tq=1  ReactP=0
  Power Equation Wind Turbine (PQ Model)13 : microgridLibrary/Power Equation Wind Turbine (PQ Model)  Commented=on  Unom=15  Umax=25  Umin=5  Pselect=Simple Cubic Power  Vrms=230*1e3  Fnom=60  rp=5  Cp=16/27  rho=1.225  Pnom=300*1e6  Uvec=[1:1:30]  Pvec=[0,0,0,0,21359.3750000000,58193.5000000000,104316.125000000,157104.500000000,213935.875000000,272187.500000000,329236.625000000,382460.500000000,429236.375000000,466941.500000000,492953.125000000,500000,500000,500000,500000,500000,500000,500000,500000,500000,500000,0,0,0,0,0]  Tp=0.1  Tq=1  ReactP=0
  Power Equation Wind Turbine (PQ Model)8 : microgridLibrary/Power Equation Wind Turbine (PQ Model)  Commented=on  Unom=15  Umax=25  Umin=5  Pselect=Simple Cubic Power  Vrms=230*1e3  Fnom=60  rp=5  Cp=16/27  rho=1.225  Pnom=60*1e6  Uvec=[1:1:30]  Pvec=[0,0,0,0,21359.3750000000,58193.5000000000,104316.125000000,157104.500000000,213935.875000000,272187.500000000,329236.625000000,382460.500000000,429236.375000000,466941.500000000,492953.125000000,500000,500000,500000,500000,500000,500000,500000,500000,500000,500000,0,0,0,0,0]  Tp=0.1  Tq=1  ReactP=0
  Power Equation Wind Turbine (PQ Model)9 : microgridLibrary/Power Equation Wind Turbine (PQ Model)  Commented=on  Unom=15  Umax=25  Umin=5  Pselect=Simple Cubic Power  Vrms=230*1e3  Fnom=60  rp=5  Cp=16/27  rho=1.225  Pnom=60*1e6  Uvec=[1:1:30]  Pvec=[0,0,0,0,21359.3750000000,58193.5000000000,104316.125000000,157104.500000000,213935.875000000,272187.500000000,329236.625000000,382460.500000000,429236.375000000,466941.500000000,492953.125000000,500000,500000,500000,500000,500000,500000,500000,500000,500000,500000,0,0,0,0,0]  Tp=0.1  Tq=1  ReactP=0
  Scope1 : Scope  Commented=on
  TVI4 : powerlib/Elements/Three-Phase Transformer (Two Windings)  Commented=on  Winding1Connection=Yg  Winding2Connection=Yg  CoreType=Three single-phase transformers  SetSaturation=off  Hysteresis=off  DataFile='hysteresis'  SetInitialFlux=off  Measurements=None  UNITS=pu  NominalPower=[ 400*1e6 , 60 ]  Winding1=[ 20*1e3, 1e-6 , 0 ]  Winding2=[ 230*1e3, 0 , 17 ]  Rm=500  Lm=500  L0=0.5  Saturation=[ 0,0 ; 0.0024,1.2 ; 1.0,1.52 ]  InitialFluxes=[ 0.8 , -0.8 , 0.7 ]  BreakLoop=off  DiscreteSolver=Trapezoidal iterative  DataType=off  TransfoNumber=0
  Trafo 14 : powerlib/Elements/Three-Phase Transformer (Two Windings)  Winding1Connection=Delta (D1)  Winding2Connection=Yg  CoreType=Three single-phase transformers  SetSaturation=off  Hysteresis=off  DataFile='hysteresis'  SetInitialFlux=off  Measurements=None  UNITS=pu  NominalPower=[ 400e6 60 ]  Winding1="[138e3 0.0023  0.0839]"  Winding2=[230e3 0.0023 0.0839]  Rm=500  Lm=500  L0=0.5  Saturation="[ 0,0  ;  0.005,1.2  ;  1.0,1.4 ]"  InitialFluxes=[ 0.8 , -0.8 , 0.7 ]  BreakLoop=off  DiscreteSolver=Trapezoidal iterative  DataType=off  TransfoNumber=0
      settings: SourceProductName=Simscape Electrical
  Trafo 15 : powerlib/Elements/Three-Phase Transformer (Two Windings)  Winding1Connection=Delta (D1)  Winding2Connection=Yg  CoreType=Three single-phase transformers  SetSaturation=off  Hysteresis=off  DataFile='hysteresis'  SetInitialFlux=off  Measurements=None  UNITS=pu  NominalPower=[ 450 60 ]  Winding1="[138e3 0.0023  0.0839]"  Winding2=[230e3 0.0023 0.0839]  Rm=500  Lm=500  L0=0.5  Saturation="[ 0,0  ;  0.005,1.2  ;  1.0,1.4 ]"  InitialFluxes=[ 0.8 , -0.8 , 0.7 ]  BreakLoop=off  DiscreteSolver=Trapezoidal iterative  DataType=off  TransfoNumber=0
      settings: SourceProductName=Simscape Electrical
  Trafo 16 : powerlib/Elements/Three-Phase Transformer (Two Windings)  Winding1Connection=Delta (D1)  Winding2Connection=Yg  CoreType=Three single-phase transformers  SetSaturation=off  Hysteresis=off  DataFile='hysteresis'  SetInitialFlux=off  Measurements=None  UNITS=pu  NominalPower=[ 500e6 60 ]  Winding1="[138e3 0.0023  0.0839]"  Winding2=[230e3 0.0023 0.0839]  Rm=500  Lm=500  L0=0.5  Saturation="[ 0,0  ;  0.005,1.2  ;  1.0,1.4 ]"  InitialFluxes=[ 0.8 , -0.8 , 0.7 ]  BreakLoop=off  DiscreteSolver=Trapezoidal iterative  DataType=off  TransfoNumber=0
      settings: SourceProductName=Simscape Electrical
  Trafo 17 : powerlib/Elements/Three-Phase Transformer (Two Windings)  Winding1Connection=Delta (D1)  Winding2Connection=Yg  CoreType=Three single-phase transformers  SetSaturation=off  Hysteresis=off  DataFile='hysteresis'  SetInitialFlux=off  Measurements=None  UNITS=pu  NominalPower=[ 410e6 60 ]  Winding1="[138e3 0.0023  0.0839]"  Winding2=[230e3 0.0023 0.0839]  Rm=500  Lm=500  L0=0.5  Saturation="[ 0,0  ;  0.005,1.2  ;  1.0,1.4 ]"  InitialFluxes=[ 0.8 , -0.8 , 0.7 ]  BreakLoop=off  DiscreteSolver=Trapezoidal iterative  DataType=off  TransfoNumber=0
      settings: SourceProductName=Simscape Electrical
  "Trafo 7 " : powerlib/Elements/Three-Phase Transformer (Two Windings)  Winding1Connection=Delta (D1)  Winding2Connection=Yg  CoreType=Three single-phase transformers  SetSaturation=off  Hysteresis=off  DataFile='hysteresis'  SetInitialFlux=off  Measurements=None  UNITS=pu  NominalPower=[ 400e6 60 ]  Winding1="[138e3 0.0023  0.0839]"  Winding2=[230e3 0.0023 0.0839]  Rm=500  Lm=500  L0=0.5  Saturation="[ 0,0  ;  0.005,1.2  ;  1.0,1.4 ]"  InitialFluxes=[ 0.8 , -0.8 , 0.7 ]  BreakLoop=off  DiscreteSolver=Trapezoidal iterative  DataType=off  TransfoNumber=0
      settings: SourceProductName=Simscape Electrical
  V01_vo : ComplexToMagnitudeAngle
  V02_vo : ComplexToMagnitudeAngle
  V13_vo : ComplexToMagnitudeAngle
  V15_vo : ComplexToMagnitudeAngle
  V16_vo1 : ComplexToMagnitudeAngle
  V18_vo1 : ComplexToMagnitudeAngle
  V21_vo1 : ComplexToMagnitudeAngle
  V22_vo1 : ComplexToMagnitudeAngle
  V23_vo2 : ComplexToMagnitudeAngle
  powergui : powerlib/powergui  Priority=1  SimulationMode=Phasor  SampleTime=10e-6  frequency=60  Iterations=50  frequencyindice=60  Pbase=100e6  ErrMax=0.0001  UnitsV=kV  UnitsW=MW  buscounter=0  FunctionMessages=off  echomessages=off  EnableUseOfTLC=off  CurrentSourceSwitches=off  DisableSnubberDevices=off  DisableRonSwitches=off  DisableVfSwitches=off  DisplayEquations=off  AutomaticDiscreteSolvers=off  SolverType=Tustin  Interpol=off  ExternalGateDelay=off  methode=off  Ts=100  x0status=blocks  SPID=off  SwTol=0  HookPort=off  NonlinearTolerance=1e-4  nMaxIteration=100  ContinueOnMaxIteration=off  RestoreLinks=warning  ResistiveCurrentMeasurement=off  Frange=[0:2:500]  Ylog=off  Xlog=on  ShowGrid=off  save=off  variable=ZData  structure=0  ZoomFFT=off  StartTime=0.0  cycles=1  DisplayStyle=1  fundamental=60  FreqAxis=off  MaxFrequency=1000  frequencyindicesteady=1  RmsSteady=1  display=off
      settings: SourceProductName=Simscape Electrical
  pu to Hz{,1..13} (14 alike) : Gain  Gain=60
  w_gen [Hz] : Scope
  Out1 : Outport  SignalName=w011
  Out2 : Outport  Port=2  SignalName=w021
  Out3 : Outport  Port=3  SignalName=w131
  Out4 : Outport  Port=4  SignalName=w132
  Out5 : Outport  Port=5  SignalName=w152
  Out6 : Outport  Port=6  SignalName=w161
  Out7 : Outport  Port=7  SignalName=w181
  Out8 : Outport  Port=8  SignalName=w211
  Out9 : Outport  Port=9  SignalName=w216
  Out19 : Outport  Port=10  SignalName=w221
  Out10 : Outport  Port=11  SignalName=v01
  Out11 : Outport  Port=12  SignalName=v02
  Out12 : Outport  Port=13  SignalName=v13
  Out13 : Outport  Port=14  SignalName=v15
  Out14 : Outport  Port=15  SignalName=v16
  Out15 : Outport  Port=16  SignalName=v18
  Out16 : Outport  Port=17  SignalName=v21
  Out17 : Outport  Port=18  SignalName=v22
  Out18 : Outport  Port=19  SignalName=v23
  Out20 : Outport  Port=20  SignalName=w023
  Out21 : Outport  Port=21  SignalName=w231
  Out22 : Outport  Port=22  SignalName=w234
  tag scope: PSSmodel=global
  wires:
  PSS model/1 -> [PSSmodel]
  [w011] -> Mux/1
  [w021] -> Mux/2
  [w152] -> Mux/6
  [w132] -> Mux/5
  [w131] -> Mux/4
  pu to Hz/1 -> w_gen [Hz]/1
  Mux/1 -> pu to Hz/1
  [w221] -> Mux/11
  [Vabc_22] -> Gain7/1
  [Vabc_21] -> Gain6/1
  [Vabc_18] -> Gain3/1
  [Vabc_01] -> Gain/1
  [Vabc_16] -> Gain2/1
  [Vabc_23] -> Gain8/1
  [w011] -> pu to Hz1/1
  pu to Hz1/1 -> Out1/1
  [w021] -> pu to Hz2/1
  pu to Hz2/1 -> Out2/1
  [w131] -> pu to Hz3/1
  pu to Hz3/1 -> Out3/1
  [w132] -> pu to Hz4/1
  pu to Hz4/1 -> Out4/1
  [w152] -> pu to Hz5/1
  pu to Hz5/1 -> Out5/1
  [w161] -> pu to Hz6/1
  pu to Hz6/1 -> Out6/1
  [w181] -> pu to Hz7/1
  pu to Hz7/1 -> Out7/1
  [w211] -> pu to Hz8/1
  pu to Hz8/1 -> Out8/1
  [w216] -> pu to Hz9/1
  pu to Hz9/1 -> Out9/1
  [w221] -> pu to Hz10/1
  pu to Hz10/1 -> Out19/1
  [Vabc_15] -> Gain5/1
  Gain4/1 -> V13_vo/1
  [Vabc_13] -> Gain4/1
  V01_vo/1 -> Out10/1, CPS mag/1
  [Vabc_02] -> Gain1/1
  V13_vo/1 -> Out12/1, CPS mag/3
  V02_vo/1 -> Out11/1, CPS mag/2
  Gain/1 -> V01_vo/1
  V15_vo/1 -> Out13/1, CPS mag/4
  Gain5/1 -> V15_vo/1
  Gain1/1 -> V02_vo/1
  Gain3/1 -> V18_vo1/1
  Gain2/1 -> V16_vo1/1
  Gain7/1 -> V22_vo1/1
  Gain6/1 -> V21_vo1/1
  Gain8/1 -> V23_vo2/1
  V16_vo1/1 -> Out14/1, CPS mag/5
  V18_vo1/1 -> Out15/1, CPS mag/6
  V21_vo1/1 -> Out16/1, CPS mag/7
  V22_vo1/1 -> Out17/1, CPS mag/8
  V23_vo2/1 -> Out18/1, CPS mag/9
  Constant9/1 -> Power Equation Wind Turbine (PQ Model)8/1
  Constant8/1 -> Power Equation Wind Turbine (PQ Model)8/2
  Constant11/1 -> Power Equation Wind Turbine (PQ Model)9/1
  Constant10/1 -> Power Equation Wind Turbine (PQ Model)9/2
  Constant13/1 -> Power Equation Wind Turbine (PQ Model)10/2
  Constant14/1 -> Power Equation Wind Turbine (PQ Model)10/1
  Constant19/1 -> Power Equation Wind Turbine (PQ Model)11/2
  Constant20/1 -> Power Equation Wind Turbine (PQ Model)11/1
  Power Equation Wind Turbine (PQ Model)12/1 -> Scope1/1
  Constant26/1 -> Power Equation Wind Turbine (PQ Model)12/1
  Constant25/1 -> Power Equation Wind Turbine (PQ Model)12/2
  Constant27/1 -> Power Equation Wind Turbine (PQ Model)13/2
  Constant28/1 -> Power Equation Wind Turbine (PQ Model)13/1
  [w023] -> Mux/3
  [w161] -> Mux/7
  [w181] -> Mux/8
  [w211] -> Mux/9
  [w216] -> Mux/10
  [w231] -> Mux/12
  [w234] -> Mux/13
  [w023] -> pu to Hz11/1
  pu to Hz11/1 -> Out20/1
  pu to Hz12/1 -> Out21/1
  [w231] -> pu to Hz12/1
  pu to Hz13/1 -> Out22/1
  [w234] -> pu to Hz13/1
  connections:
  181/LConn3 -- Power Equation Wind Turbine (PQ Model)10/LConn3 -- Base Load 5/LConn3 -- 1/RConn3 -- 2/RConn3 -- Bus18/RConn1
  Bus18/RConn3 -- Load Flow Bus/LConn1 -- 181/LConn1 -- Power Equation Wind Turbine (PQ Model)10/LConn1 -- Base Load 5/LConn1 -- 1/RConn1 -- 2/RConn1
  Bus18/RConn2 -- 2/RConn2 -- 181/LConn2 -- Power Equation Wind Turbine (PQ Model)10/LConn2 -- Base Load 5/LConn2 -- 1/RConn2
  Bus18/LConn3 -- 30/LConn1
  Bus18/LConn1 -- 30/LConn3
  Bus17/RConn3 -- 4/RConn1 -- 30/RConn1
  Bus17/RConn2 -- 4/RConn2 -- 30/RConn2
  Bus17/RConn1 -- 30/RConn3 -- 4/RConn3
  Bus16/RConn1 -- 5/RConn3 -- 28/RConn3 -- 161/LConn3
  Bus16/RConn3 -- Load Flow Bus11/LConn1 -- 161/LConn1 -- 5/RConn1 -- 28/RConn1
  Bus16/RConn2 -- 5/RConn2 -- 28/RConn2 -- 161/LConn2
  28/LConn1 -- Bus17/LConn3
  Bus17/LConn2 -- 28/LConn2
  Bus21/RConn3 -- 3/RConn1 -- 1/LConn1 -- Load Flow Bus3/LConn1 -- 216/LConn1 -- Power Equation Wind Turbine (PQ Model)9/LConn1 -- 211/LConn1 -- 212/LConn1 -- 213/LConn1 -- 214/LConn1 -- 215/LConn1 -- Base Load 18/LConn1 -- 2/LConn1
  Bus21/RConn2 -- 3/RConn2 -- 1/LConn2 -- 216/LConn2 -- Power Equation Wind Turbine (PQ Model)9/LConn2 -- 211/LConn2 -- 212/LConn2 -- 213/LConn2 -- 214/LConn2 -- 215/LConn2 -- Base Load 18/LConn2 -- 2/LConn2
  Bus21/RConn1 -- Base Load 18/LConn3 -- 213/LConn3 -- 212/LConn3 -- Power Equation Wind Turbine (PQ Model)9/LConn3 -- 211/LConn3 -- 216/LConn3 -- 214/LConn3 -- 215/LConn3 -- 1/LConn3 -- 3/RConn3 -- 2/LConn3
  Bus22/RConn1 -- 221/LConn3 -- 3/LConn3
  Bus22/RConn2 -- 221/LConn2 -- 3/LConn2
  221/LConn1 -- Load Flow Bus6/LConn1 -- Bus22/RConn3 -- 3/LConn1
  Bus21/LConn3 -- 25/LConn1 -- 43/RConn1
  Bus21/LConn2 -- 43/RConn2 -- 25/LConn2
  Bus21/LConn1 -- 25/LConn3 -- 43/RConn3
  17/RConn1 -- 25/RConn1 -- 43/LConn1 -- 154/LConn1 -- 153/LConn1 -- 152/LConn1 -- Power Equation Wind Turbine (PQ Model)12/LConn1 -- 151/LConn1 -- Load Flow Bus5/LConn1 -- Bus15/LConn3
  17/RConn2 -- 25/RConn2 -- 43/LConn2 -- Power Equation Wind Turbine (PQ Model)12/LConn2 -- 154/LConn2 -- 153/LConn2 -- 152/LConn2 -- 151/LConn2 -- Bus15/LConn2
  17/RConn3 -- 25/RConn3 -- Power Equation Wind Turbine (PQ Model)12/LConn3 -- 154/LConn3 -- 153/LConn3 -- 152/LConn3 -- 151/LConn3 -- Bus15/LConn1 -- 43/LConn3
  Base Load 17/LConn1 -- L-49-2/LConn1 -- 14/RConn1 -- Bus16/LConn3
  L-49-2/LConn2 -- Base Load 17/LConn2 -- 14/RConn2 -- Bus16/LConn2
  Bus16/LConn1 -- 14/RConn3 -- Base Load 17/LConn3 -- L-49-2/LConn3
  Base Load 16/LConn1 -- L-49-2/RConn1 -- Bus15/RConn3
  Base Load 16/LConn2 -- L-49-2/RConn2 -- Bus15/RConn2
  Base Load 16/LConn3 -- Bus15/RConn1 -- L-49-2/RConn3
  Bus22/LConn3 -- 4/LConn1
  4/LConn2 -- Bus22/LConn2
  Bus22/LConn1 -- 4/LConn3
  Bus19/LConn3 -- 5/LConn1
  5/LConn2 -- Bus19/LConn2
  5/LConn3 -- Bus19/LConn1
  7/RConn1 -- 6/RConn1 -- Bus19/RConn3 -- Base Load 1/LConn1
  7/RConn2 -- 6/RConn2 -- Bus19/RConn2 -- Base Load 1/LConn2
  Bus19/RConn1 -- 7/RConn3 -- 6/RConn3 -- Base Load 1/LConn3
  Bus20/LConn3 -- 7/LConn1 -- 6/LConn1
  Bus20/LConn2 -- 7/LConn2 -- 6/LConn2
  Bus20/LConn1 -- 7/LConn3 -- 6/LConn3
  Bus23/LConn3 -- 11/RConn1 -- 10/RConn1 -- 9/RConn1 -- 8/RConn1
  10/RConn2 -- 8/RConn2 -- 9/RConn2 -- 11/RConn2 -- Bus23/LConn2
  Bus23/LConn1 -- 10/RConn3 -- 8/RConn3 -- 9/RConn3 -- 11/RConn3
  Base Load 2/LConn2 -- 9/LConn2 -- 8/LConn2 -- Bus20/RConn2
  Base Load 2/LConn3 -- 9/LConn3 -- 8/LConn3 -- Bus20/RConn1
  Base Load 14/LConn3 -- 134/LConn3 -- 132/LConn3 -- 131/LConn3 -- Bus13/RConn1 -- 133/LConn3 -- 135/LConn3 -- Power Equation Wind Turbine (PQ Model)13/LConn3
  Base Load 14/LConn1 -- Load Flow Bus10/LConn1 -- 131/LConn1 -- 132/LConn1 -- Bus13/RConn3 -- 133/LConn1 -- 134/LConn1 -- 135/LConn1 -- Power Equation Wind Turbine (PQ Model)13/LConn1
  Base Load 14/LConn2 -- 131/LConn2 -- 132/LConn2 -- Bus13/RConn2 -- 133/LConn2 -- 134/LConn2 -- 135/LConn2 -- Power Equation Wind Turbine (PQ Model)13/LConn2
  Base Load 15/LConn1 -- 15/RConn1 -- Bus14/LConn3
  Base Load 15/LConn2 -- 15/RConn2 -- Bus14/LConn2
  Base Load 15/LConn3 -- Bus14/LConn1 -- 15/RConn3
  Bus11/RConn3 -- 15/LConn1 -- 16/LConn1
  16/LConn3 -- Bus11/RConn1 -- 15/LConn3
  Bus11/RConn2 -- 16/LConn2 -- 15/LConn2
  Bus13/LConn3 -- 16/RConn1 -- 12/RConn1 -- 11/LConn1
  Bus13/LConn2 -- 16/RConn2 -- 12/RConn2 -- 11/LConn2
  Bus13/LConn1 -- 16/RConn3 -- 12/RConn3 -- 11/LConn3
  14/LConn1 -- Bus14/RConn3
  14/LConn2 -- Bus14/RConn2
  14/LConn3 -- Bus14/RConn1
  Trafo 15/RConn1 -- Bus12/LConn3 -- 12/LConn1 -- 10/LConn1
  Trafo 15/RConn2 -- 12/LConn2 -- Bus12/LConn2 -- 10/LConn2
  Trafo 15/RConn3 -- 10/LConn3 -- 12/LConn3 -- Bus12/LConn1
  Bus24/LConn3 -- "Trafo 7 "/RConn1
  Bus24/LConn2 -- "Trafo 7 "/RConn2
  "Trafo 7 "/RConn3 -- Bus24/LConn1
  Bus3/LConn3 -- 19/LConn1 -- 18/RConn1
  Bus3/LConn2 -- 19/LConn2 -- 18/RConn2
  19/LConn3 -- Bus3/LConn1 -- 18/RConn3
  23/LConn1 -- 18/LConn1 -- Bus1/RConn3 -- 24/LConn1
  23/LConn2 -- 18/LConn2 -- 24/LConn2 -- Bus1/RConn2
  Bus1/RConn1 -- 24/LConn3 -- 23/LConn3 -- 18/LConn3
  Trafo 14/RConn1 -- Trafo 16/RConn1 -- Bus11/LConn3
  Trafo 14/RConn2 -- Trafo 16/RConn2 -- Bus11/LConn2
  Trafo 14/RConn3 -- Trafo 16/RConn3 -- Bus11/LConn1
  Bus9/RConn3 -- Trafo 15/LConn1 -- Trafo 14/LConn1
  Bus9/RConn2 -- Trafo 15/LConn2 -- Trafo 14/LConn2
  Bus9/RConn1 -- Trafo 15/LConn3 -- Trafo 14/LConn3
  "Trafo 7 "/LConn1 -- Base Load 12/LConn1 -- Bus3/RConn3
  "Trafo 7 "/LConn2 -- Base Load 12/LConn2 -- Bus3/RConn2
  "Trafo 7 "/LConn3 -- Base Load 12/LConn3 -- Bus3/RConn1
  Bus5/LConn3 -- 23/RConn1 -- Base Load 13/LConn1
  Base Load 13/LConn2 -- 23/RConn2 -- Bus5/LConn2
  Base Load 13/LConn3 -- 23/RConn3 -- Bus5/LConn1
  Bus4/RConn3 -- 21/LConn1 -- 22/LConn1
  Bus4/RConn2 -- 22/LConn2 -- 21/LConn2
  Bus4/RConn1 -- 22/LConn3 -- 21/LConn3
  26/LConn1 -- 22/RConn1 -- 24/RConn1 -- Bus2/RConn3
  22/RConn2 -- 26/LConn2 -- 24/RConn2 -- Bus2/RConn2
  22/RConn3 -- 26/LConn3 -- 24/RConn3 -- Bus2/RConn1
  26/RConn1 -- 27/RConn1 -- Bus6/RConn1
  Bus6/RConn2 -- 27/RConn2 -- 26/RConn2
  27/RConn3 -- 26/RConn3 -- Bus6/RConn3
  29/LConn1 -- 21/RConn1 -- 19/RConn1 -- Bus9/LConn3 -- Base Load 7/LConn1
  Base Load 7/LConn2 -- 29/LConn2 -- 21/RConn2 -- 19/RConn2 -- Bus9/LConn2
  Bus9/LConn1 -- 29/LConn3 -- 21/RConn3 -- 19/RConn3 -- Base Load 7/LConn3
  Bus5/RConn3 -- 20/LConn1
  Bus5/RConn2 -- 20/LConn2
  Bus5/RConn1 -- 20/LConn3
  31/LConn1 -- 27/LConn1 -- 20/RConn1 -- Base Load 8/LConn1 -- Bus10/LConn3
  Bus10/LConn2 -- 20/RConn2 -- Base Load 8/LConn2 -- 31/LConn2 -- 27/LConn2
  31/LConn3 -- 27/LConn3 -- Base Load 8/LConn3 -- 20/RConn3 -- Bus10/LConn1
  Bus10/RConn3 -- Trafo 16/LConn1 -- Trafo 17/LConn1
  Bus10/RConn2 -- Trafo 16/LConn2 -- Trafo 17/LConn2
  Bus10/RConn1 -- Trafo 16/LConn3 -- Trafo 17/LConn3
  Trafo 17/RConn1 -- Bus12/RConn3
  Trafo 17/RConn2 -- Bus12/RConn2
  Trafo 17/RConn3 -- Bus12/RConn1
  Base Load 3/LConn1 -- Bus6/LConn1
  Base Load 3/LConn2 -- Bus6/LConn2
  Bus6/LConn3 -- Base Load 3/LConn3
  Base Load 4/LConn1 -- TVI4/RConn1 -- Bus8/RConn3
  Bus8/RConn2 -- TVI4/RConn2 -- Base Load 4/LConn2
  Base Load 4/LConn3 -- TVI4/RConn3 -- Bus8/RConn1
  Bus8/LConn3 -- 32/RConn1 -- 29/RConn1 -- 31/RConn1
  Bus8/LConn2 -- 32/RConn2 -- 31/RConn2 -- 29/RConn2
  Bus8/LConn1 -- 32/RConn3 -- 31/RConn3 -- 29/RConn3
  32/LConn1 -- Bus7/RConn3
  32/LConn2 -- Bus7/RConn2
  Bus7/RConn1 -- 32/LConn3
  Base Load 6/LConn1 -- Bus4/LConn3
  Base Load 6/LConn2 -- Bus4/LConn2
  Base Load 6/LConn3 -- Bus4/LConn1
  Power Equation Wind Turbine (PQ Model)11/LConn2 -- Bus7/LConn2 -- Base Load 9/LConn2
  Bus7/LConn1 -- Power Equation Wind Turbine (PQ Model)11/LConn3 -- Base Load 9/LConn3
  Bus7/LConn3 -- Load Flow Bus2/LConn1 -- Base Load 9/LConn1 -- Power Equation Wind Turbine (PQ Model)11/LConn1
  Bus2/LConn3 -- "021 "/LConn1 -- 022/LConn1 -- Load Flow Bus1/LConn1 -- 026/LConn1 -- 025/LConn1 -- Base Load 11/LConn1 -- 024/LConn1 -- 023/LConn1
  Base Load 10/LConn2 -- 013/LConn2 -- 011/LConn2 -- Bus1/LConn2 -- 012/LConn2
  013/LConn3 -- Base Load 10/LConn3 -- 012/LConn3 -- 011/LConn3 -- Bus1/LConn1
  17/LConn1 -- Bus24/RConn3
  17/LConn2 -- Bus24/RConn2
  Bus24/RConn1 -- 17/LConn3
  Base Load 2/LConn1 -- 9/LConn1 -- 8/LConn1 -- Bus20/RConn3
  Bus17/LConn1 -- 28/LConn3
  30/LConn2 -- Bus18/LConn2
  231/LConn1 -- Load Flow Bus7/LConn1 -- Bus23/RConn3 -- Power Equation Wind Turbine (PQ Model)8/LConn1 -- 232/LConn1 -- 233/LConn1 -- 234/LConn1 -- 235/LConn1 -- 236/LConn1
  231/LConn2 -- 236/LConn2 -- 233/LConn2 -- Bus23/RConn2 -- Power Equation Wind Turbine (PQ Model)8/LConn2 -- 232/LConn2 -- 234/LConn2 -- 235/LConn2
  231/LConn3 -- 236/LConn3 -- 235/LConn3 -- 234/LConn3 -- 233/LConn3 -- 232/LConn3 -- Bus23/RConn1 -- Power Equation Wind Turbine (PQ Model)8/LConn3
  Bus2/LConn1 -- 022/LConn3 -- 024/LConn3 -- 025/LConn3 -- 026/LConn3 -- Base Load 11/LConn3 -- 023/LConn3 -- "021 "/LConn3
  Base Load 11/LConn2 -- 026/LConn2 -- 025/LConn2 -- 022/LConn2 -- "021 "/LConn2 -- Bus2/LConn2 -- 023/LConn2 -- 024/LConn2
  3-Phase Dynamic Load3/LConn1 -- TVI4/LConn1
  3-Phase Dynamic Load3/LConn2 -- TVI4/LConn2
  TVI4/LConn3 -- 3-Phase Dynamic Load3/LConn3
  Load Flow Bus4/LConn1 -- Base Load 10/LConn1 -- 013/LConn1 -- 012/LConn1 -- Bus1/LConn3 -- 011/LConn1
